simulink model "Sample594"  (R2021b)
settings: Solver=VariableStepAuto  StartTime=0.0  StopTime=10.0  RelTol=1e-3
undefined symbols (not defined in the file): DiscIntNeverNeededParam, magnitude, Newton, Raphson
libraries: simulink x402, pid_lib x98
(part 8 of 14)

== system Sample594/cfblk12/cfblk9/cfblk5/cfblk9 ==
  cfblk1 : Inport
  cfblk14 : Inport  Port=2
  cfblk15 : Inport  Port=3
  cfblk10 : Assignment  DiagnosticForDimensions=Warning  IndexOptions=Index vector (dialog)  Indices=1  OutputSizes=1
  cfblk11 : Constant  Value=[-794911285.649197]  SampleTime=1
  cfblk12 : Constant  Value=[-113984455.118114]  SampleTime=1
  cfblk13 : Constant  Value=[597938276.331210]  SampleTime=1
  cfblk16 : Delay
  cfblk3 : UnitDelay  SampleTime=-1  HasFrameUpgradeWarning=on
  cfblk4 : Delay  DelayLengthSource=Input port
      settings: InputPortMap=u0,p1
  cfblk5 : simulink/Discrete/Difference  ICPrevInput=0.0  OutMin=[]  OutMax=[]  OutDataTypeStr=Inherit: Inherit via back propagation  OutDataType=fixdt(1, 16)  OutScaling=2^-10  DoSatur=off
  cfblk6 : UnitDelay  SampleTime=-1  HasFrameUpgradeWarning=on
  cfblk7 : DiscreteIntegrator  SampleTime=-1  ICPrevOutput=DiscIntNeverNeededParam  ICPrevScaledInput=DiscIntNeverNeededParam
  cfblk8 : Math  Operator=rem  SaturateOnIntegerOverflow=on
  cfblk9 : simulink/Math Operations/Slider Gain  gain=1  low=0  high=2
  cfblk2 : Outport
  wires:
  cfblk5/1 -> cfblk7/1
  cfblk3/1 -> cfblk9/1
  cfblk11/1 -> cfblk6/1
  cfblk1/1 -> cfblk8/1
  cfblk7/1 -> cfblk2/1
  cfblk12/1 -> cfblk10/1
  cfblk6/1 -> cfblk8/2
  cfblk14/1 -> cfblk10/2
  cfblk8/1 -> cfblk4/1
  cfblk10/1 -> cfblk5/1
  cfblk15/1 -> cfblk4/2
  cfblk9/1 -> cfblk16/1
  cfblk16/1 -> cfblk3/1

== system Sample594/cfblk12/cfblk9/cfblk6/cfblk6 ==
  cfblk1 : Inport
  cfblk7 : Inport  Port=2
  cfblk3 : DiscreteFir
  cfblk4 : Assignment  DiagnosticForDimensions=Warning  IndexOptions=Index vector (dialog)  Indices=1  OutputSizes=1
  cfblk5 : Sqrt  SaturateOnIntegerOverflow=on
  cfblk6 : Constant  Value=[-543936318.988298]  SampleTime=1
  cfblk8 : Delay
  cfblk2 : Outport
  wires:
  cfblk6/1 -> cfblk2/1
  cfblk3/1 -> cfblk5/1
  cfblk1/1 -> cfblk4/1
  cfblk7/1 -> cfblk4/2
  cfblk5/1 -> cfblk8/1
  cfblk8/1 -> cfblk3/1

== system Sample594/cfblk12/cfblk9/cfblk6/cfblk7 ==
  cfblk1 : Inport
  cfblk7 : Inport  Port=2
  cfblk8 : Inport  Port=3
  cfblk9 : Inport  Port=4
  cfblk10 : Inport  Port=5
  cfblk3 : Gain  Gain=[572937926.758752]
  cfblk4 : Bias  Bias=[905543510.378754]
  cfblk5 : Product
  cfblk6 : Constant  Value=[-979519378.910522]  SampleTime=1
  cfblk2 : Outport
  wires:
  cfblk10/1 -> cfblk5/1
  cfblk8/1 -> cfblk4/1
  cfblk7/1 -> cfblk2/1
  cfblk6/1 -> cfblk5/2
  cfblk1/1 -> cfblk3/1

== system Sample594/cfblk12/cfblk9/cfblk6/cfblk8 ==
  cfblk1 : Inport
  cfblk16 : Inport  Port=2
  cfblk10 : simulink/Math Operations/Slider Gain  gain=1  low=0  high=2
  cfblk11 : ComplexToMagnitudeAngle
  cfblk12 : Squeeze
  cfblk13 : Sqrt  Operator=rSqrt  AlgorithmType=Newton-Raphson  SaturateOnIntegerOverflow=on
  cfblk14 : Constant  Value=[356714615.940462]  SampleTime=1
  cfblk15 : Constant  Value=[-873089521.906120]  SampleTime=1
  cfblk18 : Delay
  cfblk3 : DiscreteFilter
  cfblk4 : simulink/Discrete/Transfer Fcn First Order  PoleZ=0.95  ICPrevOutput=0.0  DoSatur=off
  cfblk5 : DiscreteZeroPole  Poles=[0 0.5]  Gain=1  SampleTime=-1
  cfblk6 : Delay  ShowEnablePort=on
      settings: InputPortMap=u0,e6
  cfblk7 : simulink/Discrete/Transfer Fcn First Order  PoleZ=0.95  ICPrevOutput=0.0  DoSatur=off
  cfblk8 : Sum  Inputs=|++
  cfblk9 : DotProduct  InputSameDT=on  OutDataTypeStr=Inherit: Inherit via internal rule
  cfblk2 : Outport
  cfblk17 : Outport  Port=2
  wires:
  cfblk13/1 -> cfblk4/1
  cfblk4/1 -> cfblk11/1
  cfblk1/1 -> cfblk7/1
  cfblk7/1 -> cfblk3/1
  cfblk12/1 -> cfblk5/1
  cfblk9/1 -> cfblk8/2
  cfblk11/1 -> cfblk2/1
  cfblk11/2 -> cfblk17/1
  cfblk15/1 -> cfblk10/1
  cfblk8/1 -> cfblk6/1
  cfblk3/1 -> cfblk9/1
  cfblk16/1 -> cfblk13/1
  cfblk14/1 -> cfblk12/1
  cfblk5/1 -> cfblk6/2
  cfblk10/1 -> cfblk9/2
  cfblk6/1 -> cfblk18/1
  cfblk18/1 -> cfblk8/1

== system Sample594/cfblk12/cfblk9/cfblk7/cfblk7 ==
  cfblk1 : Inport
  cfblk7 : Inport  Port=2
  cfblk8 : Inport  Port=3
  cfblk9 : Inport  Port=4
  cfblk3 : Sum  Inputs=+-
  cfblk4 : Sum  Inputs=-+
  cfblk5 : MinMax  Inputs=2
  cfblk6 : Constant  Value=[114627535.775119]  SampleTime=1
  cfblk2 : Outport
  cfblk10 : Outport  Port=2
  wires:
  cfblk7/1 -> cfblk3/1
  cfblk9/1 -> cfblk2/1
  cfblk3/1 -> cfblk5/1
  cfblk1/1 -> cfblk5/2
  cfblk6/1 -> cfblk4/1
  cfblk5/1 -> cfblk4/2
  cfblk4/1 -> cfblk10/1
  cfblk8/1 -> cfblk3/2

== system Sample594/cfblk12/cfblk9/cfblk7/cfblk8 ==
  cfblk1 : Inport
  cfblk11 : Inport  Port=2
  cfblk12 : Inport  Port=3
  cfblk13 : Inport  Port=4
  cfblk10 : DotProduct  InputSameDT=on  OutDataTypeStr=Inherit: Inherit via internal rule
  cfblk3 : DiscreteIntegrator  SampleTime=-1  ICPrevOutput=DiscIntNeverNeededParam  ICPrevScaledInput=DiscIntNeverNeededParam
  cfblk4 : DiscreteStateSpace  SampleTime=-1
  cfblk5 : simulink/Discrete/Transfer Fcn Real Zero  ZeroZ=0.75  ICPrevInput=0.0  DoSatur=off
      settings: SourceProductBaseCode=SL
  cfblk6 : Product
  cfblk7 : UnaryMinus
  cfblk8 : Sin  TimeSource=Use external signal  SampleTime=0
  cfblk9 : PermuteDimensions
  cfblk2 : Outport
  cfblk14 : Outport  Port=2
  wires:
  cfblk13/1 -> cfblk14/1
  cfblk11/1 -> cfblk10/1
  cfblk12/1 -> cfblk9/1
  cfblk6/1 -> cfblk2/1
  cfblk9/1 -> cfblk3/1
  cfblk3/1 -> cfblk8/1
  cfblk10/1 -> cfblk5/1
  cfblk7/1 -> cfblk10/2
  cfblk5/1 -> cfblk4/1
  cfblk4/1 -> cfblk6/1
  cfblk8/1 -> cfblk6/2
  cfblk1/1 -> cfblk7/1

== system Sample594/cfblk12/cfblk9/cfblk7/cfblk9 ==
  cfblk1 : Inport
  cfblk12 : Inport  Port=2
  cfblk13 : Inport  Port=3
  cfblk10 : Constant  Value=[554921363.762607]  SampleTime=1
  cfblk11 : Constant  Value=[554197841.356145]  SampleTime=1
  cfblk15 : Delay
  cfblk16 : Delay
  cfblk3 : Delay
  cfblk4 : Sqrt  Operator=rSqrt  AlgorithmType=Newton-Raphson  SaturateOnIntegerOverflow=on
  cfblk5 : Squeeze
  cfblk6 : Product
  cfblk7 : UnaryMinus
  cfblk8 : Rounding
  cfblk9 : Constant  Value=[-430584521.529058]  SampleTime=1
  cfblk2 : Outport
  cfblk14 : Outport  Port=2
  wires:
  cfblk13/1 -> cfblk2/1
  cfblk12/1 -> cfblk8/1
  cfblk9/1 -> cfblk14/1
  cfblk1/1 -> cfblk4/1
  cfblk3/1 -> cfblk7/1
  cfblk8/1 -> cfblk6/1
  cfblk5/1 -> cfblk6/2
  cfblk7/1 -> cfblk15/1
  cfblk15/1 -> cfblk3/1
  cfblk6/1 -> cfblk16/1
  cfblk16/1 -> cfblk5/1

== system Sample594/cfblk5/cfblk8/cfblk7/cfblk10 ==
  cfblk1 : Inport
  cfblk5 : Inport  Port=2
  cfblk6 : Inport  Port=3
  cfblk3 : DiscreteStateSpace
  cfblk4 : Delay  SampleTime=1
  cfblk2 : Outport
  cfblk7 : Outport  Port=2
  wires:
  cfblk3/1 -> cfblk7/1
  cfblk5/1 -> cfblk2/1
  cfblk6/1 -> cfblk3/1
  cfblk1/1 -> cfblk4/1

== system Sample594/cfblk5/cfblk8/cfblk7/cfblk11 ==
  cfblk1 : Inport
  cfblk8 : Inport  Port=2
  cfblk9 : Inport  Port=3
  cfblk10 : Inport  Port=4
  cfblk11 : Inport  Port=5
  cfblk12 : Inport  Port=6
  cfblk13 : Inport  Port=7
  cfblk17 : Delay  SampleTime=1
  cfblk3 : DiscreteStateSpace
  cfblk4 : ComplexToMagnitudeAngle
  cfblk5 : Bias  Bias=[-448982168.775191]
  cfblk6 : Sum  Inputs=|++
  cfblk7 : Bias  Bias=[-341245710.573488]
  cfblk2 : Outport
  cfblk14 : Outport  Port=2
  cfblk15 : Outport  Port=3
  cfblk16 : Outport  Port=4
  wires:
  cfblk8/1 -> cfblk5/1
  cfblk5/1 -> cfblk2/1
  cfblk1/1 -> cfblk14/1
  cfblk4/1 -> cfblk16/1
  cfblk9/1 -> cfblk7/1
  cfblk11/1 -> cfblk4/1
  cfblk13/1 -> cfblk15/1
  cfblk7/1 -> cfblk6/1
  cfblk3/1 -> cfblk6/2
  cfblk6/1 -> cfblk17/1
  cfblk17/1 -> cfblk3/1

== system Sample594/cfblk5/cfblk8/cfblk7/cfblk12 ==
  cfblk1 : Inport
  cfblk7 : Inport  Port=2
  cfblk8 : Inport  Port=3
  cfblk9 : Inport  Port=4
  cfblk10 : Inport  Port=5
  cfblk3 : simulink/Math Operations/Slider Gain  gain=1  low=0  high=2
  cfblk4 : Product  Inputs=**
  cfblk5 : Sum  Inputs=|++
  cfblk6 : Constant  Value=[231752368.860097]  SampleTime=1
  cfblk2 : Outport
  cfblk11 : Outport  Port=2
  wires:
  cfblk7/1 -> cfblk11/1
  cfblk4/1 -> cfblk2/1
  cfblk5/1 -> cfblk4/1
  cfblk6/1 -> cfblk3/1
  cfblk10/1 -> cfblk5/1
  cfblk9/1 -> cfblk4/2
  cfblk8/1 -> cfblk5/2

== system Sample594/cfblk5/cfblk8/cfblk7/cfblk13 ==
  cfblk1 : Inport
  cfblk14 : Inport  Port=2
  cfblk10 : Gain  Gain=[27691866.060482]
  cfblk11 : UnaryMinus
  cfblk12 : MinMax  Function=max  Inputs=3
  cfblk13 : Constant  Value=[379580006.162565]  SampleTime=1
  cfblk15 : Delay  SampleTime=1
  cfblk16 : Delay  SampleTime=1
  cfblk17 : Delay  SampleTime=1
  cfblk3 : DiscreteIntegrator  ICPrevOutput=DiscIntNeverNeededParam  ICPrevScaledInput=DiscIntNeverNeededParam
  cfblk4 : simulink/Discrete/Tapped Delay  vinit=0.0  samptime=-1  NumDelays=1  DelayOrder=Oldest  includeCurrent=off
  cfblk5 : simulink/Discrete/Transfer Fcn Lead or Lag  PoleZ=0.95  ZeroZ=0.75  ICPrevOutput=0.0  ICPrevInput=0.0  DoSatur=off
      settings: SourceProductBaseCode=SL
  cfblk6 : Delay  ShowEnablePort=on  SampleTime=1
      settings: InputPortMap=u0,e6
  cfblk7 : Product  Inputs=**
  cfblk8 : Bias  Bias=[-450394797.310045]
  cfblk9 : ComplexToRealImag
  cfblk2 : Outport
  wires:
  cfblk6/1 -> cfblk4/1
  cfblk11/1 -> cfblk8/1
  cfblk12/1 -> cfblk10/1
  cfblk5/1 -> cfblk7/1
  cfblk4/1 -> cfblk9/1
  cfblk10/1 -> cfblk5/1, cfblk16/1
  cfblk9/1 -> cfblk2/1
  cfblk1/1 -> cfblk11/1
  cfblk8/1 -> cfblk12/1
  cfblk14/1 -> cfblk7/2
  cfblk3/1 -> cfblk6/1
  cfblk13/1 -> cfblk6/2
  cfblk7/1 -> cfblk15/1
  cfblk15/1 -> cfblk12/2
  cfblk16/1 -> cfblk12/3
  cfblk9/2 -> cfblk17/1
  cfblk17/1 -> cfblk3/1

== system Sample594/cfblk5/cfblk8/cfblk7/cfblk17 ==
  cfblk1 : Inport
  cfblk10 : Inport  Port=2
  cfblk11 : Inport  Port=3
  cfblk12 : Inport  Port=4
  Action Port : ActionPort  ActionPortLabel=if(u1 >= 0)
  cfblk3 : Polyval  Coefs=[ +2.081618890e-019, -1.441693666e-014, +4.719686976e-010, -8.536869453e-006, +1.621573104e-001, -8.087801117e+001 ]
  cfblk4 : UnaryMinus
  cfblk5 : DotProduct  InputSameDT=on  OutDataTypeStr=Inherit: Inherit via internal rule
  cfblk6 : MinMax  Function=max  Inputs=2
  cfblk7 : Rounding
  cfblk8 : Constant  Value=[138414329.532610]  SampleTime=1
  cfblk9 : Constant  Value=[747672156.969024]  SampleTime=1
  cfblk2 : Outport
  cfblk13 : Outport  Port=2
  cfblk14 : Outport  Port=3
  cfblk15 : Outport  Port=4
  wires:
  cfblk9/1 -> cfblk3/1
  cfblk4/1 -> cfblk13/1
  cfblk11/1 -> cfblk5/1
  cfblk7/1 -> cfblk5/2
  cfblk10/1 -> cfblk6/1
  cfblk3/1 -> cfblk15/1
  cfblk1/1 -> cfblk14/1
  cfblk6/1 -> cfblk2/1
  cfblk8/1 -> cfblk6/2
  cfblk5/1 -> cfblk4/1
  cfblk12/1 -> cfblk7/1

== system Sample594/cfblk5/cfblk8/cfblk7/cfblk18 ==
  cfblk1 : Inport
  Action Port : ActionPort  ActionPortLabel=else
  cfblk3 : DiscreteStateSpace  SampleTime=-1
  cfblk4 : Signum
  cfblk5 : Abs
  cfblk6 : Constant  Value=[-798494818.476831]  SampleTime=1
  cfblk2 : Outport
  cfblk7 : Outport  Port=2
  wires:
  cfblk3/1 -> cfblk4/1
  cfblk6/1 -> cfblk2/1
  cfblk4/1 -> cfblk7/1
  cfblk1/1 -> cfblk3/1, cfblk5/1

== system Sample594/cfblk5/cfblk8/cfblk7/cfblk9 ==
  cfblk1 : Inport
  cfblk15 : Inport  Port=2
  cfblk16 : Inport  Port=3
  cfblk17 : Inport  Port=4
  cfblk10 : Math  Operator=conj  SaturateOnIntegerOverflow=on
  cfblk11 : simulink/Math Operations/Slider Gain  gain=1  low=0  high=2
  cfblk12 : Abs
  cfblk13 : Constant  Value=[207080615.983424]  SampleTime=1
  cfblk14 : Constant  Value=[514869977.372286]  SampleTime=1
  cfblk18 : Delay  SampleTime=1
  cfblk3 : Delay  DelayLengthSource=Input port  SampleTime=1
      settings: InputPortMap=u0,p1
  cfblk4 : Delay  DelayLengthSource=Input port  SampleTime=1
      settings: InputPortMap=u0,p1
  cfblk5 : DiscreteFilter  SampleTime=1
  cfblk6 : Sum  Inputs=+
  cfblk7 : Trigonometry
  cfblk8 : Rounding
  cfblk9 : Sin  TimeSource=Use external signal  SampleTime=0
  cfblk2 : Outport
  wires:
  cfblk15/1 -> cfblk2/1
  cfblk8/1 -> cfblk3/1
  cfblk14/1 -> cfblk9/1
  cfblk1/1 -> cfblk6/1
  cfblk7/1 -> cfblk5/1
  cfblk13/1 -> cfblk7/1
  cfblk16/1 -> cfblk4/1
  cfblk6/1 -> cfblk3/2
  cfblk4/1 -> cfblk12/1
  cfblk5/1 -> cfblk10/1
  cfblk17/1 -> cfblk11/1
  cfblk10/1 -> cfblk8/1
  cfblk12/1 -> cfblk18/1
  cfblk18/1 -> cfblk4/2

== system Sample594/cfblk5/cfblk8/cfblk8/cfblk10 ==
  cfblk1 : Inport
  cfblk3 : DiscreteZeroPole  Poles=[0 0.5]  Gain=1
  cfblk4 : DiscreteTransferFcn  SampleTime=1
  cfblk5 : Delay  SampleTime=1
  cfblk6 : Sqrt  Operator=rSqrt  AlgorithmType=Newton-Raphson  SaturateOnIntegerOverflow=on
  cfblk7 : Trigonometry
  cfblk2 : Outport
  wires:
  cfblk7/1 -> cfblk5/1
  cfblk4/1 -> cfblk2/1
  cfblk5/1 -> cfblk3/1
  cfblk6/1 -> cfblk7/1
  cfblk1/1 -> cfblk6/1
  cfblk3/1 -> cfblk4/1

== system Sample594/cfblk5/cfblk8/cfblk8/cfblk13 ==
  cfblk1 : Inport
  cfblk7 : Inport  Port=2
  cfblk8 : Inport  Port=3
  cfblk9 : Inport  Port=4
  Action Port : ActionPort  ActionPortLabel=if(u1 >= 0)
  cfblk3 : Delay  ShowEnablePort=on
      settings: InputPortMap=u0,e6
  cfblk4 : simulink/Discrete/Transfer Fcn First Order  PoleZ=0.95  ICPrevOutput=0.0  DoSatur=off
  cfblk5 : Abs
  cfblk6 : Sum  Inputs=+-
  cfblk2 : Outport
  cfblk10 : Outport  Port=2
  cfblk11 : Outport  Port=3
  wires:
  cfblk1/1 -> cfblk5/1
  cfblk5/1 -> cfblk6/1
  cfblk4/1 -> cfblk2/1
  cfblk8/1 -> cfblk3/1
  cfblk7/1 -> cfblk4/1
  cfblk3/1 -> cfblk6/2, cfblk10/1
  cfblk6/1 -> cfblk11/1
  cfblk9/1 -> cfblk3/2

== system Sample594/cfblk5/cfblk8/cfblk8/cfblk14 ==
  cfblk1 : Inport
  cfblk8 : Inport  Port=2
  Action Port : ActionPort  ActionPortLabel=else
  cfblk10 : Delay
  cfblk3 : DiscreteFilter
  cfblk4 : Math  Operator=pow  SaturateOnIntegerOverflow=on
  cfblk5 : MinMax  Inputs=2
  cfblk6 : Sin  TimeSource=Use external signal  SampleTime=0
  cfblk7 : Constant  Value=[22445580.202978]  SampleTime=1
  cfblk2 : Outport
  cfblk9 : Outport  Port=2
  wires:
  cfblk7/1 -> cfblk5/1
  cfblk8/1 -> cfblk6/1
  cfblk1/1 -> cfblk5/2
  cfblk4/1 -> cfblk3/1
  cfblk6/1 -> cfblk2/1
  cfblk5/1 -> cfblk4/2, cfblk9/1
  cfblk3/1 -> cfblk10/1
  cfblk10/1 -> cfblk4/1

== system Sample594/cfblk5/cfblk8/cfblk8/cfblk8 ==
  cfblk1 : Inport
  cfblk7 : Inport  Port=2
  cfblk3 : Delay  SampleTime=1
  cfblk4 : pid_lib/PID Controller (2DOF)  Controller=PID  Form=Parallel  TimeDomain=Discrete-time  UseExternalTs=off  SampleTime=1  IntegratorMethod=Forward Euler  FilterMethod=Forward Euler  ControllerParametersSource=internal  P=1  I=1  D=0  UseFilter=on  N=100  b=1  c=1  TunerSelectOption=Transfer Function Based (PID Tuner App)  InitialConditionSource=internal  InitialConditionForIntegrator=0  InitialConditionForFilter=0  DifferentiatorICPrevScaledInput=0  ExternalReset=none  TrackingMode=off  Kt=1  LimitOutput=off  SatLimitsSource=internal  UpperSaturationLimit=inf  LowerSaturationLimit=-inf  LinearizeAsGain=off  AntiWindupMode=none  Kb=1  POutMin=[]  POutMax=[]  IOutMin=[]  IOutMax=[]  DOutMin=[]  DOutMax=[]  NOutMin=[]  NOutMax=[]  bOutMin=[]  bOutMax=[]  cOutMin=[]  cOutMax=[]  SumOutMin=[]  SumOutMax=[]  SaturationOutMin=[]  SaturationOutMax=[]  PParamMin=[]  PParamMax=[]  IParamMin=[]  IParamMax=[]  DParamMin=[]  DParamMax=[]  NParamMin=[]  NParamMax=[]  bParamMin=[]  bParamMax=[]  cParamMin=[]  cParamMax=[]  KbParamMin=[]  KbParamMax=[]  KtParamMin=[]  KtParamMax=[]  KbOutMin=[]  KbOutMax=[]  KtOutMin=[]  KtOutMax=[]  IntegratorOutMin=[]  IntegratorOutMax=[]  FilterOutMin=[]  FilterOutMax=[]  SumI1OutMin=[]  SumI1OutMax=[]  SumI2OutMin=[]  SumI2OutMax=[]  SumI3OutMin=[]  SumI3OutMax=[]  SumI4OutMin=[]  SumI4OutMax=[]  SumDOutMin=[]  SumDOutMax=[]  Sum1OutMin=[]  Sum1OutMax=[]  Sum2OutMin=[]  Sum2OutMax=[]  Sum3OutMin=[]  Sum3OutMax=[]  DifferentiatorOutMin=[]  DifferentiatorOutMax=[]  FilterDiffOutCoefMin=[]  FilterDiffOutCoefMax=[]  ReciprocalOutMin=[]  ReciprocalOutMax=[]  SumDenOutMin=[]  SumDenOutMax=[]  SumNumOutMin=[]  SumNumOutMax=[]  DivideOutMin=[]  DivideOutMax=[]  UdiffTsProdOutMin=[]  UdiffTsProdOutMax=[]  NTsProdOutMin=[]  NTsProdOutMax=[]  UintegralTsProdOutMin=[]  UintegralTsProdOutMax=[]  UngainTsProdOutMin=[]  UngainTsProdOutMax=[]  IntegratorContinuousStateAttributes=''  IntegratorStateMustResolveToSignalObject=off  IntegratorRTWStateStorageClass=Auto  FilterContinuousStateAttributes=''  FilterStateMustResolveToSignalObject=off  FilterRTWStateStorageClass=Auto  ParallelPVariant=InternalParameters  IdealPVariant=Disabled  IVariant=InternalParameters  DVariant=InternalParameters  bVariant=InternalParameters  cVariant=InternalParameters  IntegratorVariant=Discrete  SatVariant=Disabled  AWVariant=Passthrough  PCopyVariant=Disabled  TRVariant=Disabled  FdbkBlocksVariant=Forward  IdealPFdbkVariant=Disabled  SatFdbkVariant=Disabled  DerivativeFilterVariant=ForwardEulerFilter  NVariant=InternalParameters  NCopyVariant=Disabled  FilterICVariant=InternalICsFilter  IntegratorICVariant=InternalICs  ExternalResetVariant=Disabled  TRSumVariant=Passthrough  SumFdbkVariant=Disabled  SumVariant=Sum_PID  TsampFilterVariant=InternalTs  TsampNgainVariant=Passthrough  TsampIntegralVariant=Passthrough  ExternalSaturationOutDataTypeStr=Inherit: Same as second input
      settings: SourceProductBaseCode=SL
  cfblk5 : simulink/Math Operations/MinMax Running Resettable  Function=min  vinit=0.0
  cfblk6 : Constant  Value=[-209440082.700214]  SampleTime=1
  cfblk8 : Delay  SampleTime=1
  cfblk2 : Outport
  wires:
  cfblk7/1 -> cfblk3/1
  cfblk6/1 -> cfblk5/1
  cfblk3/1 -> cfblk2/1
  cfblk4/1 -> cfblk5/2
  cfblk1/1 -> cfblk4/2
  cfblk5/1 -> cfblk8/1
  cfblk8/1 -> cfblk4/1

== system Sample594/cfblk5/cfblk8/cfblk8/cfblk9 ==
  cfblk1 : Inport
  cfblk12 : Inport  Port=2
  cfblk13 : Inport  Port=3
  cfblk14 : Inport  Port=4
  cfblk10 : Product  Inputs=**
  cfblk11 : Sum  Inputs=+-
  cfblk3 : DiscreteIntegrator  ICPrevOutput=DiscIntNeverNeededParam  ICPrevScaledInput=DiscIntNeverNeededParam
  cfblk4 : DiscreteTransferFcn  SampleTime=1
  cfblk5 : pid_lib/PID Controller (2DOF)  Controller=PID  Form=Parallel  TimeDomain=Discrete-time  UseExternalTs=off  SampleTime=1  IntegratorMethod=Forward Euler  FilterMethod=Forward Euler  ControllerParametersSource=internal  P=1  I=1  D=0  UseFilter=on  N=100  b=1  c=1  TunerSelectOption=Transfer Function Based (PID Tuner App)  InitialConditionSource=internal  InitialConditionForIntegrator=0  InitialConditionForFilter=0  DifferentiatorICPrevScaledInput=0  ExternalReset=none  TrackingMode=off  Kt=1  LimitOutput=off  SatLimitsSource=internal  UpperSaturationLimit=inf  LowerSaturationLimit=-inf  LinearizeAsGain=off  AntiWindupMode=none  Kb=1  POutMin=[]  POutMax=[]  IOutMin=[]  IOutMax=[]  DOutMin=[]  DOutMax=[]  NOutMin=[]  NOutMax=[]  bOutMin=[]  bOutMax=[]  cOutMin=[]  cOutMax=[]  SumOutMin=[]  SumOutMax=[]  SaturationOutMin=[]  SaturationOutMax=[]  PParamMin=[]  PParamMax=[]  IParamMin=[]  IParamMax=[]  DParamMin=[]  DParamMax=[]  NParamMin=[]  NParamMax=[]  bParamMin=[]  bParamMax=[]  cParamMin=[]  cParamMax=[]  KbParamMin=[]  KbParamMax=[]  KtParamMin=[]  KtParamMax=[]  KbOutMin=[]  KbOutMax=[]  KtOutMin=[]  KtOutMax=[]  IntegratorOutMin=[]  IntegratorOutMax=[]  FilterOutMin=[]  FilterOutMax=[]  SumI1OutMin=[]  SumI1OutMax=[]  SumI2OutMin=[]  SumI2OutMax=[]  SumI3OutMin=[]  SumI3OutMax=[]  SumI4OutMin=[]  SumI4OutMax=[]  SumDOutMin=[]  SumDOutMax=[]  Sum1OutMin=[]  Sum1OutMax=[]  Sum2OutMin=[]  Sum2OutMax=[]  Sum3OutMin=[]  Sum3OutMax=[]  DifferentiatorOutMin=[]  DifferentiatorOutMax=[]  FilterDiffOutCoefMin=[]  FilterDiffOutCoefMax=[]  ReciprocalOutMin=[]  ReciprocalOutMax=[]  SumDenOutMin=[]  SumDenOutMax=[]  SumNumOutMin=[]  SumNumOutMax=[]  DivideOutMin=[]  DivideOutMax=[]  UdiffTsProdOutMin=[]  UdiffTsProdOutMax=[]  NTsProdOutMin=[]  NTsProdOutMax=[]  UintegralTsProdOutMin=[]  UintegralTsProdOutMax=[]  UngainTsProdOutMin=[]  UngainTsProdOutMax=[]  IntegratorContinuousStateAttributes=''  IntegratorStateMustResolveToSignalObject=off  IntegratorRTWStateStorageClass=Auto  FilterContinuousStateAttributes=''  FilterStateMustResolveToSignalObject=off  FilterRTWStateStorageClass=Auto  ParallelPVariant=InternalParameters  IdealPVariant=Disabled  IVariant=InternalParameters  DVariant=InternalParameters  bVariant=InternalParameters  cVariant=InternalParameters  IntegratorVariant=Discrete  SatVariant=Disabled  AWVariant=Passthrough  PCopyVariant=Disabled  TRVariant=Disabled  FdbkBlocksVariant=Forward  IdealPFdbkVariant=Disabled  SatFdbkVariant=Disabled  DerivativeFilterVariant=ForwardEulerFilter  NVariant=InternalParameters  NCopyVariant=Disabled  FilterICVariant=InternalICsFilter  IntegratorICVariant=InternalICs  ExternalResetVariant=Disabled  TRSumVariant=Passthrough  SumFdbkVariant=Disabled  SumVariant=Sum_PID  TsampFilterVariant=InternalTs  TsampNgainVariant=Passthrough  TsampIntegralVariant=Passthrough  ExternalSaturationOutDataTypeStr=Inherit: Same as second input
      settings: SourceProductBaseCode=SL
  cfblk6 : Abs
  cfblk7 : Abs
  cfblk8 : Squeeze
  cfblk9 : DotProduct  InputSameDT=on  OutDataTypeStr=Inherit: Inherit via internal rule
  cfblk2 : Outport
  wires:
  cfblk13/1 -> cfblk8/1
  cfblk9/1 -> cfblk10/1
  cfblk6/1 -> cfblk9/1
  cfblk4/1 -> cfblk3/1
  cfblk12/1 -> cfblk4/1
  cfblk14/1 -> cfblk11/1
  cfblk3/1 -> cfblk10/2
  cfblk5/1 -> cfblk6/1
  cfblk1/1 -> cfblk5/1
  cfblk11/1 -> cfblk5/2
  cfblk8/1 -> cfblk7/1
  cfblk7/1 -> cfblk9/2, cfblk11/2
  cfblk10/1 -> cfblk2/1

== system Sample594/cfblk6/cfblk10/cfblk6/cfblk10 ==
  cfblk1 : Inport
  cfblk5 : Inport  Port=2
  cfblk6 : Inport  Port=3
  cfblk3 : pid_lib/PID Controller  Controller=PID  Form=Parallel  TimeDomain=Discrete-time  UseExternalTs=off  SampleTime=1  IntegratorMethod=Forward Euler  FilterMethod=Forward Euler  ControllerParametersSource=internal  P=1  I=1  D=0  UseFilter=on  N=100  TunerSelectOption=Transfer Function Based (PID Tuner App)  InitialConditionSource=internal  InitialConditionForIntegrator=0  InitialConditionForFilter=0  DifferentiatorICPrevScaledInput=0  ExternalReset=none  TrackingMode=off  Kt=1  LimitOutput=off  SatLimitsSource=internal  UpperSaturationLimit=inf  LowerSaturationLimit=-inf  LinearizeAsGain=off  AntiWindupMode=none  Kb=1  POutMin=[]  POutMax=[]  IOutMin=[]  IOutMax=[]  DOutMin=[]  DOutMax=[]  NOutMin=[]  NOutMax=[]  SumOutMin=[]  SumOutMax=[]  SaturationOutMin=[]  SaturationOutMax=[]  PParamMin=[]  PParamMax=[]  IParamMin=[]  IParamMax=[]  DParamMin=[]  DParamMax=[]  NParamMin=[]  NParamMax=[]  KbParamMin=[]  KbParamMax=[]  KtParamMin=[]  KtParamMax=[]  KbOutMin=[]  KbOutMax=[]  KtOutMin=[]  KtOutMax=[]  IntegratorOutMin=[]  IntegratorOutMax=[]  FilterOutMin=[]  FilterOutMax=[]  SumI1OutMin=[]  SumI1OutMax=[]  SumI2OutMin=[]  SumI2OutMax=[]  SumI3OutMin=[]  SumI3OutMax=[]  SumI4OutMin=[]  SumI4OutMax=[]  SumDOutMin=[]  SumDOutMax=[]  DifferentiatorOutMin=[]  DifferentiatorOutMax=[]  FilterDiffOutCoefMin=[]  FilterDiffOutCoefMax=[]  ReciprocalOutMin=[]  ReciprocalOutMax=[]  SumDenOutMin=[]  SumDenOutMax=[]  SumNumOutMin=[]  SumNumOutMax=[]  DivideOutMin=[]  DivideOutMax=[]  UdiffTsProdOutMin=[]  UdiffTsProdOutMax=[]  NTsProdOutMin=[]  NTsProdOutMax=[]  UintegralTsProdOutMin=[]  UintegralTsProdOutMax=[]  UngainTsProdOutMin=[]  UngainTsProdOutMax=[]  IntegratorContinuousStateAttributes=''  IntegratorStateMustResolveToSignalObject=off  IntegratorRTWStateStorageClass=Auto  FilterContinuousStateAttributes=''  FilterStateMustResolveToSignalObject=off  FilterRTWStateStorageClass=Auto  ParallelPVariant=InternalParameters  IdealPVariant=Disabled  IVariant=InternalParameters  DVariant=InternalParameters  IntegratorVariant=Discrete  SatVariant=Disabled  AWVariant=Passthrough  PCopyVariant=Disabled  TRVariant=Disabled  FdbkBlocksVariant=Forward  IdealPFdbkVariant=Disabled  SatFdbkVariant=Disabled  DerivativeFilterVariant=ForwardEulerFilter  NVariant=InternalParameters  NCopyVariant=Disabled  FilterICVariant=InternalICsFilter  IntegratorICVariant=InternalICs  ExternalResetVariant=Disabled  TRSumVariant=Passthrough  SumFdbkVariant=Disabled  SumVariant=Sum_PID  TsampFilterVariant=InternalTs  TsampNgainVariant=Passthrough  TsampIntegralVariant=Passthrough  ExternalSaturationOutDataTypeStr=Inherit: Same as second input
  cfblk4 : Sqrt  SaturateOnIntegerOverflow=on
  cfblk2 : Outport
  cfblk7 : Outport  Port=2
  wires:
  cfblk3/1 -> cfblk4/1
  cfblk5/1 -> cfblk7/1
  cfblk1/1 -> cfblk2/1
  cfblk6/1 -> cfblk3/1

== system Sample594/cfblk6/cfblk10/cfblk6/cfblk11 ==
  cfblk1 : Inport
  cfblk13 : Inport  Port=2
  cfblk14 : Inport  Port=3
  cfblk15 : Inport  Port=4
  cfblk10 : Assignment  DiagnosticForDimensions=Warning  IndexOptions=Index vector (dialog)  Indices=1  OutputSizes=1
  cfblk11 : Reshape
  cfblk12 : DotProduct  InputSameDT=on  OutDataTypeStr=Inherit: Inherit via internal rule
  cfblk{4..5,7,17} (4 alike) : Delay  SampleTime=1
  cfblk3 : DiscreteFir  SampleTime=1
  cfblk6 : Delay  ShowEnablePort=on  SampleTime=1
      settings: InputPortMap=u0,e6
  cfblk8 : DiscreteFir  SampleTime=1
  cfblk9 : Math  Operator=conj  SaturateOnIntegerOverflow=on
  cfblk2 : Outport
  cfblk16 : Outport  Port=2
  wires:
  cfblk4/1 -> cfblk7/1
  cfblk11/1 -> cfblk5/1
  cfblk8/1 -> cfblk6/1
  cfblk14/1 -> cfblk11/1
  cfblk7/1 -> cfblk10/1
  cfblk5/1 -> cfblk8/1
  cfblk3/1 -> cfblk10/2
  cfblk12/1 -> cfblk2/1
  cfblk9/1 -> cfblk6/2
  cfblk6/1 -> cfblk16/1
  cfblk1/1 -> cfblk9/1
  cfblk13/1 -> cfblk12/1
  cfblk15/1 -> cfblk4/1
  cfblk10/1 -> cfblk12/2, cfblk17/1
  cfblk17/1 -> cfblk3/1

== system Sample594/cfblk6/cfblk10/cfblk6/cfblk4 ==
  cfblk1 : Inport
  cfblk11 : Inport  Port=2
  cfblk12 : Inport  Port=3
  cfblk10 : Sum  Inputs=+-
  cfblk3 : Delay  SampleTime=1
  cfblk4 : simulink/Discrete/Transfer Fcn First Order  PoleZ=0.95  ICPrevOutput=0.0  DoSatur=off
  cfblk5 : pid_lib/PID Controller  Controller=PID  Form=Parallel  TimeDomain=Discrete-time  UseExternalTs=off  SampleTime=1  IntegratorMethod=Forward Euler  FilterMethod=Forward Euler  ControllerParametersSource=internal  P=1  I=1  D=0  UseFilter=on  N=100  TunerSelectOption=Transfer Function Based (PID Tuner App)  InitialConditionSource=internal  InitialConditionForIntegrator=0  InitialConditionForFilter=0  DifferentiatorICPrevScaledInput=0  ExternalReset=none  TrackingMode=off  Kt=1  LimitOutput=off  SatLimitsSource=internal  UpperSaturationLimit=inf  LowerSaturationLimit=-inf  LinearizeAsGain=off  AntiWindupMode=none  Kb=1  POutMin=[]  POutMax=[]  IOutMin=[]  IOutMax=[]  DOutMin=[]  DOutMax=[]  NOutMin=[]  NOutMax=[]  SumOutMin=[]  SumOutMax=[]  SaturationOutMin=[]  SaturationOutMax=[]  PParamMin=[]  PParamMax=[]  IParamMin=[]  IParamMax=[]  DParamMin=[]  DParamMax=[]  NParamMin=[]  NParamMax=[]  KbParamMin=[]  KbParamMax=[]  KtParamMin=[]  KtParamMax=[]  KbOutMin=[]  KbOutMax=[]  KtOutMin=[]  KtOutMax=[]  IntegratorOutMin=[]  IntegratorOutMax=[]  FilterOutMin=[]  FilterOutMax=[]  SumI1OutMin=[]  SumI1OutMax=[]  SumI2OutMin=[]  SumI2OutMax=[]  SumI3OutMin=[]  SumI3OutMax=[]  SumI4OutMin=[]  SumI4OutMax=[]  SumDOutMin=[]  SumDOutMax=[]  DifferentiatorOutMin=[]  DifferentiatorOutMax=[]  FilterDiffOutCoefMin=[]  FilterDiffOutCoefMax=[]  ReciprocalOutMin=[]  ReciprocalOutMax=[]  SumDenOutMin=[]  SumDenOutMax=[]  SumNumOutMin=[]  SumNumOutMax=[]  DivideOutMin=[]  DivideOutMax=[]  UdiffTsProdOutMin=[]  UdiffTsProdOutMax=[]  NTsProdOutMin=[]  NTsProdOutMax=[]  UintegralTsProdOutMin=[]  UintegralTsProdOutMax=[]  UngainTsProdOutMin=[]  UngainTsProdOutMax=[]  IntegratorContinuousStateAttributes=''  IntegratorStateMustResolveToSignalObject=off  IntegratorRTWStateStorageClass=Auto  FilterContinuousStateAttributes=''  FilterStateMustResolveToSignalObject=off  FilterRTWStateStorageClass=Auto  ParallelPVariant=InternalParameters  IdealPVariant=Disabled  IVariant=InternalParameters  DVariant=InternalParameters  IntegratorVariant=Discrete  SatVariant=Disabled  AWVariant=Passthrough  PCopyVariant=Disabled  TRVariant=Disabled  FdbkBlocksVariant=Forward  IdealPFdbkVariant=Disabled  SatFdbkVariant=Disabled  DerivativeFilterVariant=ForwardEulerFilter  NVariant=InternalParameters  NCopyVariant=Disabled  FilterICVariant=InternalICsFilter  IntegratorICVariant=InternalICs  ExternalResetVariant=Disabled  TRSumVariant=Passthrough  SumFdbkVariant=Disabled  SumVariant=Sum_PID  TsampFilterVariant=InternalTs  TsampNgainVariant=Passthrough  TsampIntegralVariant=Passthrough  ExternalSaturationOutDataTypeStr=Inherit: Same as second input
  cfblk6 : pid_lib/PID Controller  Controller=PID  Form=Parallel  TimeDomain=Discrete-time  UseExternalTs=off  SampleTime=1  IntegratorMethod=Forward Euler  FilterMethod=Forward Euler  ControllerParametersSource=internal  P=1  I=1  D=0  UseFilter=on  N=100  TunerSelectOption=Transfer Function Based (PID Tuner App)  InitialConditionSource=internal  InitialConditionForIntegrator=0  InitialConditionForFilter=0  DifferentiatorICPrevScaledInput=0  ExternalReset=none  TrackingMode=off  Kt=1  LimitOutput=off  SatLimitsSource=internal  UpperSaturationLimit=inf  LowerSaturationLimit=-inf  LinearizeAsGain=off  AntiWindupMode=none  Kb=1  POutMin=[]  POutMax=[]  IOutMin=[]  IOutMax=[]  DOutMin=[]  DOutMax=[]  NOutMin=[]  NOutMax=[]  SumOutMin=[]  SumOutMax=[]  SaturationOutMin=[]  SaturationOutMax=[]  PParamMin=[]  PParamMax=[]  IParamMin=[]  IParamMax=[]  DParamMin=[]  DParamMax=[]  NParamMin=[]  NParamMax=[]  KbParamMin=[]  KbParamMax=[]  KtParamMin=[]  KtParamMax=[]  KbOutMin=[]  KbOutMax=[]  KtOutMin=[]  KtOutMax=[]  IntegratorOutMin=[]  IntegratorOutMax=[]  FilterOutMin=[]  FilterOutMax=[]  SumI1OutMin=[]  SumI1OutMax=[]  SumI2OutMin=[]  SumI2OutMax=[]  SumI3OutMin=[]  SumI3OutMax=[]  SumI4OutMin=[]  SumI4OutMax=[]  SumDOutMin=[]  SumDOutMax=[]  DifferentiatorOutMin=[]  DifferentiatorOutMax=[]  FilterDiffOutCoefMin=[]  FilterDiffOutCoefMax=[]  ReciprocalOutMin=[]  ReciprocalOutMax=[]  SumDenOutMin=[]  SumDenOutMax=[]  SumNumOutMin=[]  SumNumOutMax=[]  DivideOutMin=[]  DivideOutMax=[]  UdiffTsProdOutMin=[]  UdiffTsProdOutMax=[]  NTsProdOutMin=[]  NTsProdOutMax=[]  UintegralTsProdOutMin=[]  UintegralTsProdOutMax=[]  UngainTsProdOutMin=[]  UngainTsProdOutMax=[]  IntegratorContinuousStateAttributes=''  IntegratorStateMustResolveToSignalObject=off  IntegratorRTWStateStorageClass=Auto  FilterContinuousStateAttributes=''  FilterStateMustResolveToSignalObject=off  FilterRTWStateStorageClass=Auto  ParallelPVariant=InternalParameters  IdealPVariant=Disabled  IVariant=InternalParameters  DVariant=InternalParameters  IntegratorVariant=Discrete  SatVariant=Disabled  AWVariant=Passthrough  PCopyVariant=Disabled  TRVariant=Disabled  FdbkBlocksVariant=Forward  IdealPFdbkVariant=Disabled  SatFdbkVariant=Disabled  DerivativeFilterVariant=ForwardEulerFilter  NVariant=InternalParameters  NCopyVariant=Disabled  FilterICVariant=InternalICsFilter  IntegratorICVariant=InternalICs  ExternalResetVariant=Disabled  TRSumVariant=Passthrough  SumFdbkVariant=Disabled  SumVariant=Sum_PID  TsampFilterVariant=InternalTs  TsampNgainVariant=Passthrough  TsampIntegralVariant=Passthrough  ExternalSaturationOutDataTypeStr=Inherit: Same as second input
  cfblk7 : Delay  SampleTime=1
  cfblk8 : Bias  Bias=[-646270231.580480]
  cfblk9 : Squeeze
  cfblk2 : Outport
  cfblk13 : Outport  Port=2
  wires:
  cfblk12/1 -> cfblk8/1
  cfblk8/1 -> cfblk4/1
  cfblk9/1 -> cfblk3/1
  cfblk1/1 -> cfblk9/1
  cfblk10/1 -> cfblk7/1
  cfblk6/1 -> cfblk10/1
  cfblk11/1 -> cfblk10/2
  cfblk4/1 -> cfblk6/1
  cfblk7/1 -> cfblk5/1
  cfblk3/1 -> cfblk13/1
  cfblk5/1 -> cfblk2/1

== system Sample594/cfblk6/cfblk10/cfblk6/cfblk5 ==
  cfblk1 : Inport
  cfblk10 : MinMax  Inputs=2
  cfblk11 : MinMax
  cfblk12 : simulink/Math Operations/Slider Gain  gain=1  low=0  high=2
  cfblk13 : Signum
  cfblk{6,15..18} (5 alike) : Delay  SampleTime=1
  cfblk3 : Delay  ShowEnablePort=on  SampleTime=1
      settings: InputPortMap=u0,e6
  cfblk4 : simulink/Discrete/Transfer Fcn Lead or Lag  PoleZ=0.95  ZeroZ=0.75  ICPrevOutput=0.0  ICPrevInput=0.0  DoSatur=off
      settings: SourceProductBaseCode=SL
  cfblk5 : simulink/Discrete/Difference  ICPrevInput=0.0  OutMin=[]  OutMax=[]  OutDataTypeStr=Inherit: Inherit via back propagation  OutDataType=fixdt(1, 16)  OutScaling=2^-10  DoSatur=off
  cfblk7 : Signum
  cfblk8 : Polyval  Coefs=[ +2.081618890e-019, -1.441693666e-014, +4.719686976e-010, -8.536869453e-006, +1.621573104e-001, -8.087801117e+001 ]
  cfblk9 : Squeeze
  cfblk2 : Outport
  cfblk14 : Outport  Port=2
  wires:
  cfblk13/1 -> cfblk12/1
  cfblk3/1 -> cfblk7/1
  cfblk4/1 -> cfblk6/1, cfblk3/2
  cfblk12/1 -> cfblk16/1, cfblk17/1
  cfblk8/1 -> cfblk3/1
  cfblk7/1 -> cfblk14/1
  cfblk10/1 -> cfblk13/1
  cfblk1/1 -> cfblk2/1
  cfblk11/1 -> cfblk8/1, cfblk18/1
  cfblk9/1 -> cfblk11/1
  cfblk5/1 -> cfblk10/1
  cfblk6/1 -> cfblk15/1
  cfblk15/1 -> cfblk4/1
  cfblk16/1 -> cfblk5/1
  cfblk17/1 -> cfblk10/2
  cfblk18/1 -> cfblk9/1

== system Sample594/cfblk6/cfblk10/cfblk6/cfblk6 ==
  cfblk1 : Inport
  cfblk13 : Inport  Port=2
  cfblk14 : Inport  Port=3
  cfblk15 : Inport  Port=4
  cfblk16 : Inport  Port=5
  cfblk17 : Inport  Port=6
  cfblk10 : Rounding
  cfblk11 : Gain  Gain=[-971098976.945693]
  cfblk12 : Constant  Value=[291546184.892133]  SampleTime=1
  cfblk3 : simulink/Discrete/Transfer Fcn Lead or Lag  PoleZ=0.95  ZeroZ=0.75  ICPrevOutput=0.0  ICPrevInput=0.0  DoSatur=off
      settings: SourceProductBaseCode=SL
  cfblk4 : DiscreteFilter  SampleTime=1
  cfblk5 : pid_lib/PID Controller (2DOF)  Controller=PID  Form=Parallel  TimeDomain=Discrete-time  UseExternalTs=off  SampleTime=1  IntegratorMethod=Forward Euler  FilterMethod=Forward Euler  ControllerParametersSource=internal  P=1  I=1  D=0  UseFilter=on  N=100  b=1  c=1  TunerSelectOption=Transfer Function Based (PID Tuner App)  InitialConditionSource=internal  InitialConditionForIntegrator=0  InitialConditionForFilter=0  DifferentiatorICPrevScaledInput=0  ExternalReset=none  TrackingMode=off  Kt=1  LimitOutput=off  SatLimitsSource=internal  UpperSaturationLimit=inf  LowerSaturationLimit=-inf  LinearizeAsGain=off  AntiWindupMode=none  Kb=1  POutMin=[]  POutMax=[]  IOutMin=[]  IOutMax=[]  DOutMin=[]  DOutMax=[]  NOutMin=[]  NOutMax=[]  bOutMin=[]  bOutMax=[]  cOutMin=[]  cOutMax=[]  SumOutMin=[]  SumOutMax=[]  SaturationOutMin=[]  SaturationOutMax=[]  PParamMin=[]  PParamMax=[]  IParamMin=[]  IParamMax=[]  DParamMin=[]  DParamMax=[]  NParamMin=[]  NParamMax=[]  bParamMin=[]  bParamMax=[]  cParamMin=[]  cParamMax=[]  KbParamMin=[]  KbParamMax=[]  KtParamMin=[]  KtParamMax=[]  KbOutMin=[]  KbOutMax=[]  KtOutMin=[]  KtOutMax=[]  IntegratorOutMin=[]  IntegratorOutMax=[]  FilterOutMin=[]  FilterOutMax=[]  SumI1OutMin=[]  SumI1OutMax=[]  SumI2OutMin=[]  SumI2OutMax=[]  SumI3OutMin=[]  SumI3OutMax=[]  SumI4OutMin=[]  SumI4OutMax=[]  SumDOutMin=[]  SumDOutMax=[]  Sum1OutMin=[]  Sum1OutMax=[]  Sum2OutMin=[]  Sum2OutMax=[]  Sum3OutMin=[]  Sum3OutMax=[]  DifferentiatorOutMin=[]  DifferentiatorOutMax=[]  FilterDiffOutCoefMin=[]  FilterDiffOutCoefMax=[]  ReciprocalOutMin=[]  ReciprocalOutMax=[]  SumDenOutMin=[]  SumDenOutMax=[]  SumNumOutMin=[]  SumNumOutMax=[]  DivideOutMin=[]  DivideOutMax=[]  UdiffTsProdOutMin=[]  UdiffTsProdOutMax=[]  NTsProdOutMin=[]  NTsProdOutMax=[]  UintegralTsProdOutMin=[]  UintegralTsProdOutMax=[]  UngainTsProdOutMin=[]  UngainTsProdOutMax=[]  IntegratorContinuousStateAttributes=''  IntegratorStateMustResolveToSignalObject=off  IntegratorRTWStateStorageClass=Auto  FilterContinuousStateAttributes=''  FilterStateMustResolveToSignalObject=off  FilterRTWStateStorageClass=Auto  ParallelPVariant=InternalParameters  IdealPVariant=Disabled  IVariant=InternalParameters  DVariant=InternalParameters  bVariant=InternalParameters  cVariant=InternalParameters  IntegratorVariant=Discrete  SatVariant=Disabled  AWVariant=Passthrough  PCopyVariant=Disabled  TRVariant=Disabled  FdbkBlocksVariant=Forward  IdealPFdbkVariant=Disabled  SatFdbkVariant=Disabled  DerivativeFilterVariant=ForwardEulerFilter  NVariant=InternalParameters  NCopyVariant=Disabled  FilterICVariant=InternalICsFilter  IntegratorICVariant=InternalICs  ExternalResetVariant=Disabled  TRSumVariant=Passthrough  SumFdbkVariant=Disabled  SumVariant=Sum_PID  TsampFilterVariant=InternalTs  TsampNgainVariant=Passthrough  TsampIntegralVariant=Passthrough  ExternalSaturationOutDataTypeStr=Inherit: Same as second input
      settings: SourceProductBaseCode=SL
  cfblk6 : Delay  SampleTime=1
  cfblk7 : simulink/Discrete/Transfer Fcn Lead or Lag  PoleZ=0.95  ZeroZ=0.75  ICPrevOutput=0.0  ICPrevInput=0.0  DoSatur=off
      settings: SourceProductBaseCode=SL
  cfblk8 : Delay  ShowEnablePort=on  SampleTime=1
      settings: InputPortMap=u0,e6
  cfblk9 : Product
  cfblk2 : Outport
  wires:
  cfblk6/1 -> cfblk11/1
  cfblk4/1 -> cfblk8/1
  cfblk12/1 -> cfblk9/1
  cfblk10/1 -> cfblk6/1
  cfblk13/1 -> cfblk9/2
  cfblk7/1 -> cfblk2/1
  cfblk14/1 -> cfblk8/2
  cfblk1/1 -> cfblk7/1
  cfblk3/1 -> cfblk10/1
  cfblk15/1 -> cfblk4/1
  cfblk9/1 -> cfblk5/1
  cfblk8/1 -> cfblk5/2
  cfblk16/1 -> cfblk3/1

== system Sample594/cfblk6/cfblk10/cfblk6/cfblk7 ==
  cfblk1 : Inport
  cfblk11 : Inport  Port=2
  cfblk12 : Inport  Port=3
  cfblk10 : Constant  Value=[875467071.398786]  SampleTime=1
  cfblk16 : Delay  SampleTime=1
  cfblk3 : simulink/Discrete/Tapped Delay  vinit=0.0  samptime=-1  NumDelays=1  DelayOrder=Oldest  includeCurrent=off
  cfblk4 : UnaryMinus
  cfblk5 : Squeeze
  cfblk6 : Product
  cfblk7 : Squeeze
  cfblk8 : Math  Operator=mod  SaturateOnIntegerOverflow=on
  cfblk9 : Product
  cfblk2 : Outport
  cfblk13 : Outport  Port=2
  cfblk14 : Outport  Port=3
  cfblk15 : Outport  Port=4
  wires:
  cfblk10/1 -> cfblk15/1
  cfblk6/1 -> cfblk13/1
  cfblk9/1 -> cfblk6/1, cfblk4/1
  cfblk11/1 -> cfblk3/1
  cfblk5/1 -> cfblk9/1
  cfblk12/1 -> cfblk14/1, cfblk6/2
  cfblk1/1 -> cfblk7/1
  cfblk8/1 -> cfblk2/1
  cfblk7/1 -> cfblk5/1
  cfblk3/1 -> cfblk8/1
  cfblk4/1 -> cfblk8/2, cfblk16/1
  cfblk16/1 -> cfblk9/2

== system Sample594/cfblk6/cfblk10/cfblk6/cfblk8 ==
  cfblk1 : Inport
  cfblk10 : UnaryMinus
  cfblk12 : Delay  SampleTime=1
  cfblk13 : Delay  SampleTime=1
  cfblk3 : pid_lib/PID Controller (2DOF)  Controller=PID  Form=Parallel  TimeDomain=Discrete-time  UseExternalTs=off  SampleTime=1  IntegratorMethod=Forward Euler  FilterMethod=Forward Euler  ControllerParametersSource=internal  P=1  I=1  D=0  UseFilter=on  N=100  b=1  c=1  TunerSelectOption=Transfer Function Based (PID Tuner App)  InitialConditionSource=internal  InitialConditionForIntegrator=0  InitialConditionForFilter=0  DifferentiatorICPrevScaledInput=0  ExternalReset=none  TrackingMode=off  Kt=1  LimitOutput=off  SatLimitsSource=internal  UpperSaturationLimit=inf  LowerSaturationLimit=-inf  LinearizeAsGain=off  AntiWindupMode=none  Kb=1  POutMin=[]  POutMax=[]  IOutMin=[]  IOutMax=[]  DOutMin=[]  DOutMax=[]  NOutMin=[]  NOutMax=[]  bOutMin=[]  bOutMax=[]  cOutMin=[]  cOutMax=[]  SumOutMin=[]  SumOutMax=[]  SaturationOutMin=[]  SaturationOutMax=[]  PParamMin=[]  PParamMax=[]  IParamMin=[]  IParamMax=[]  DParamMin=[]  DParamMax=[]  NParamMin=[]  NParamMax=[]  bParamMin=[]  bParamMax=[]  cParamMin=[]  cParamMax=[]  KbParamMin=[]  KbParamMax=[]  KtParamMin=[]  KtParamMax=[]  KbOutMin=[]  KbOutMax=[]  KtOutMin=[]  KtOutMax=[]  IntegratorOutMin=[]  IntegratorOutMax=[]  FilterOutMin=[]  FilterOutMax=[]  SumI1OutMin=[]  SumI1OutMax=[]  SumI2OutMin=[]  SumI2OutMax=[]  SumI3OutMin=[]  SumI3OutMax=[]  SumI4OutMin=[]  SumI4OutMax=[]  SumDOutMin=[]  SumDOutMax=[]  Sum1OutMin=[]  Sum1OutMax=[]  Sum2OutMin=[]  Sum2OutMax=[]  Sum3OutMin=[]  Sum3OutMax=[]  DifferentiatorOutMin=[]  DifferentiatorOutMax=[]  FilterDiffOutCoefMin=[]  FilterDiffOutCoefMax=[]  ReciprocalOutMin=[]  ReciprocalOutMax=[]  SumDenOutMin=[]  SumDenOutMax=[]  SumNumOutMin=[]  SumNumOutMax=[]  DivideOutMin=[]  DivideOutMax=[]  UdiffTsProdOutMin=[]  UdiffTsProdOutMax=[]  NTsProdOutMin=[]  NTsProdOutMax=[]  UintegralTsProdOutMin=[]  UintegralTsProdOutMax=[]  UngainTsProdOutMin=[]  UngainTsProdOutMax=[]  IntegratorContinuousStateAttributes=''  IntegratorStateMustResolveToSignalObject=off  IntegratorRTWStateStorageClass=Auto  FilterContinuousStateAttributes=''  FilterStateMustResolveToSignalObject=off  FilterRTWStateStorageClass=Auto  ParallelPVariant=InternalParameters  IdealPVariant=Disabled  IVariant=InternalParameters  DVariant=InternalParameters  bVariant=InternalParameters  cVariant=InternalParameters  IntegratorVariant=Discrete  SatVariant=Disabled  AWVariant=Passthrough  PCopyVariant=Disabled  TRVariant=Disabled  FdbkBlocksVariant=Forward  IdealPFdbkVariant=Disabled  SatFdbkVariant=Disabled  DerivativeFilterVariant=ForwardEulerFilter  NVariant=InternalParameters  NCopyVariant=Disabled  FilterICVariant=InternalICsFilter  IntegratorICVariant=InternalICs  ExternalResetVariant=Disabled  TRSumVariant=Passthrough  SumFdbkVariant=Disabled  SumVariant=Sum_PID  TsampFilterVariant=InternalTs  TsampNgainVariant=Passthrough  TsampIntegralVariant=Passthrough  ExternalSaturationOutDataTypeStr=Inherit: Same as second input
      settings: SourceProductBaseCode=SL
  cfblk4 : Product  Inputs=**
  cfblk5 : ComplexToMagnitudeAngle
  cfblk6 : simulink/Math Operations/Slider Gain  gain=1  low=0  high=2
  cfblk7 : Polyval  Coefs=[ +2.081618890e-019, -1.441693666e-014, +4.719686976e-010, -8.536869453e-006, +1.621573104e-001, -8.087801117e+001 ]
  cfblk8 : Sin  TimeSource=Use external signal  SampleTime=0
  cfblk9 : Signum
  cfblk2 : Outport
  cfblk11 : Outport  Port=2
  wires:
  cfblk8/1 -> cfblk12/1, cfblk13/1
  cfblk6/1 -> cfblk2/1
  cfblk5/1 -> cfblk3/2
  cfblk1/1 -> cfblk10/1
  cfblk9/1 -> cfblk7/1
  cfblk10/1 -> cfblk4/1
  cfblk5/2 -> cfblk11/1
  cfblk3/1 -> cfblk6/1, cfblk8/1
  cfblk4/1 -> cfblk9/1
  cfblk7/1 -> cfblk5/1
  cfblk12/1 -> cfblk3/1
  cfblk13/1 -> cfblk4/2

== system Sample594/cfblk6/cfblk10/cfblk6/cfblk9 ==
  cfblk1 : Inport
  cfblk13 : Inport  Port=2
  cfblk14 : Inport  Port=3
  cfblk15 : Inport  Port=4
  cfblk10 : Sin  TimeSource=Use external signal  SampleTime=0
  cfblk11 : UnaryMinus
  cfblk12 : Constant  Value=[242392632.367211]  SampleTime=1
  cfblk3 : Product  Inputs=**
  cfblk4 : Bias  Bias=[-997769937.162003]
  cfblk5 : Rounding
  cfblk6 : ComplexToRealImag
  cfblk7 : ComplexToRealImag
  cfblk8 : Rounding
  cfblk9 : UnaryMinus
  cfblk2 : Outport
  cfblk16 : Outport  Port=2
  cfblk17 : Outport  Port=3
  wires:
  cfblk10/1 -> cfblk4/1
  cfblk13/1 -> cfblk16/1
  cfblk11/1 -> cfblk6/1
  cfblk8/1 -> cfblk7/1
  cfblk5/1 -> cfblk2/1
  cfblk15/1 -> cfblk3/1
  cfblk12/1 -> cfblk3/2
  cfblk1/1 -> cfblk17/1
  cfblk4/1 -> cfblk5/1
  cfblk6/1 -> cfblk10/1
  cfblk6/2 -> cfblk8/1
  cfblk14/1 -> cfblk11/1
  cfblk7/1 -> cfblk9/1

== system Sample594/cfblk6/cfblk10/cfblk7/cfblk7 ==
  cfblk1 : Inport
  cfblk6 : Inport  Port=2
  cfblk3 : DiscreteTransferFcn  SampleTime=1
  cfblk4 : simulink/Discrete/Transfer Fcn Lead or Lag  PoleZ=0.95  ZeroZ=0.75  ICPrevOutput=0.0  ICPrevInput=0.0  DoSatur=off
      settings: SourceProductBaseCode=SL
  cfblk5 : UnitDelay  HasFrameUpgradeWarning=on
  cfblk2 : Outport
  cfblk7 : Outport  Port=2
  cfblk8 : Outport  Port=3
  wires:
  cfblk4/1 -> cfblk5/1, cfblk3/1
  cfblk5/1 -> cfblk7/1
  cfblk6/1 -> cfblk2/1
  cfblk1/1 -> cfblk4/1
  cfblk3/1 -> cfblk8/1

== system Sample594/cfblk6/cfblk10/cfblk7/cfblk8 ==
  cfblk1 : Inport
  cfblk10 : Product
  cfblk11 : Sum  Inputs=--
  cfblk12 : PermuteDimensions
  cfblk13 : Product  Inputs=*
  cfblk14 : Sin  TimeSource=Use external signal  SampleTime=0
  cfblk15 : Constant  Value=[-832231158.363719]  SampleTime=1
  cfblk16 : Delay  SampleTime=1
  cfblk17 : Delay  SampleTime=1
  cfblk18 : Delay  SampleTime=1
  cfblk3 : pid_lib/PID Controller  Controller=PID  Form=Parallel  TimeDomain=Discrete-time  UseExternalTs=off  SampleTime=1  IntegratorMethod=Forward Euler  FilterMethod=Forward Euler  ControllerParametersSource=internal  P=1  I=1  D=0  UseFilter=on  N=100  TunerSelectOption=Transfer Function Based (PID Tuner App)  InitialConditionSource=internal  InitialConditionForIntegrator=0  InitialConditionForFilter=0  DifferentiatorICPrevScaledInput=0  ExternalReset=none  TrackingMode=off  Kt=1  LimitOutput=off  SatLimitsSource=internal  UpperSaturationLimit=inf  LowerSaturationLimit=-inf  LinearizeAsGain=off  AntiWindupMode=none  Kb=1  POutMin=[]  POutMax=[]  IOutMin=[]  IOutMax=[]  DOutMin=[]  DOutMax=[]  NOutMin=[]  NOutMax=[]  SumOutMin=[]  SumOutMax=[]  SaturationOutMin=[]  SaturationOutMax=[]  PParamMin=[]  PParamMax=[]  IParamMin=[]  IParamMax=[]  DParamMin=[]  DParamMax=[]  NParamMin=[]  NParamMax=[]  KbParamMin=[]  KbParamMax=[]  KtParamMin=[]  KtParamMax=[]  KbOutMin=[]  KbOutMax=[]  KtOutMin=[]  KtOutMax=[]  IntegratorOutMin=[]  IntegratorOutMax=[]  FilterOutMin=[]  FilterOutMax=[]  SumI1OutMin=[]  SumI1OutMax=[]  SumI2OutMin=[]  SumI2OutMax=[]  SumI3OutMin=[]  SumI3OutMax=[]  SumI4OutMin=[]  SumI4OutMax=[]  SumDOutMin=[]  SumDOutMax=[]  DifferentiatorOutMin=[]  DifferentiatorOutMax=[]  FilterDiffOutCoefMin=[]  FilterDiffOutCoefMax=[]  ReciprocalOutMin=[]  ReciprocalOutMax=[]  SumDenOutMin=[]  SumDenOutMax=[]  SumNumOutMin=[]  SumNumOutMax=[]  DivideOutMin=[]  DivideOutMax=[]  UdiffTsProdOutMin=[]  UdiffTsProdOutMax=[]  NTsProdOutMin=[]  NTsProdOutMax=[]  UintegralTsProdOutMin=[]  UintegralTsProdOutMax=[]  UngainTsProdOutMin=[]  UngainTsProdOutMax=[]  IntegratorContinuousStateAttributes=''  IntegratorStateMustResolveToSignalObject=off  IntegratorRTWStateStorageClass=Auto  FilterContinuousStateAttributes=''  FilterStateMustResolveToSignalObject=off  FilterRTWStateStorageClass=Auto  ParallelPVariant=InternalParameters  IdealPVariant=Disabled  IVariant=InternalParameters  DVariant=InternalParameters  IntegratorVariant=Discrete  SatVariant=Disabled  AWVariant=Passthrough  PCopyVariant=Disabled  TRVariant=Disabled  FdbkBlocksVariant=Forward  IdealPFdbkVariant=Disabled  SatFdbkVariant=Disabled  DerivativeFilterVariant=ForwardEulerFilter  NVariant=InternalParameters  NCopyVariant=Disabled  FilterICVariant=InternalICsFilter  IntegratorICVariant=InternalICs  ExternalResetVariant=Disabled  TRSumVariant=Passthrough  SumFdbkVariant=Disabled  SumVariant=Sum_PID  TsampFilterVariant=InternalTs  TsampNgainVariant=Passthrough  TsampIntegralVariant=Passthrough  ExternalSaturationOutDataTypeStr=Inherit: Same as second input
  cfblk4 : DiscreteFir  SampleTime=1
  cfblk5 : Delay  ShowEnablePort=on  SampleTime=1
      settings: InputPortMap=u0,e6
  cfblk6 : simulink/Discrete/Transfer Fcn Lead or Lag  PoleZ=0.95  ZeroZ=0.75  ICPrevOutput=0.0  ICPrevInput=0.0  DoSatur=off
      settings: SourceProductBaseCode=SL
  cfblk7 : Delay  DelayLengthSource=Input port  SampleTime=1
      settings: InputPortMap=u0,p1
  cfblk8 : Assignment  DiagnosticForDimensions=Warning  IndexOptions=Index vector (dialog)  Indices=1  OutputSizes=1
  cfblk9 : Sum  Inputs=|++
  cfblk2 : Outport
  wires:
  cfblk6/1 -> cfblk4/1
  cfblk11/1 -> cfblk12/1, cfblk17/1
  cfblk5/1 -> cfblk14/1
  cfblk15/1 -> cfblk8/1
  cfblk3/1 -> cfblk6/1, cfblk18/1
  cfblk14/1 -> cfblk8/2
  cfblk7/1 -> cfblk11/2
  cfblk4/1 -> cfblk10/1, cfblk10/2
  cfblk1/1 -> cfblk2/1, cfblk13/1
  cfblk9/1 -> cfblk3/1
  cfblk13/1 -> cfblk7/1, cfblk9/1
  cfblk12/1 -> cfblk5/1
  cfblk10/1 -> cfblk5/2
  cfblk8/1 -> cfblk16/1
  cfblk16/1 -> cfblk11/1
  cfblk17/1 -> cfblk7/2
  cfblk18/1 -> cfblk9/2
